simulink model "mdlref_basic"  (Simulink 7.8)
settings: Solver=FixedStepDiscrete  SolverMode=SingleTasking  StartTime=0.0  StopTime=10.0  FixedStep=0.1  RelTol=1e-3
settings Model: Creator=The MathWorks Inc.  LastModifiedBy=itoy  ExtModeAutoUpdateStatusClock=off
settings DataIOCC: SaveFormat=StructureWithTime  SignalLoggingName=logsOut
settings OptimizationCC: InlineParams=on  InlineInvariantSignals=on  InitFltsAndDblsToZero=on
settings DebuggingCC: SaveWithParameterizedLinksMsg=none  CheckExecutionContextPreStartOutputMsg=on  CheckExecutionContextRuntimeOutputMsg=on  SolverPrmCheckMsg=none  MultiTaskDSMMsg=warning  MultiTaskCondExecSysMsg=none  SigSpecEnsureSampleTimeMsg=none  FcnCallInpInsideContextMsg=Use local settings  StrictBusMsg=ErrorOnBusTreatedAsVector
settings HardwareCC: TargetHWDeviceType=32-bit Generic
settings ModelReferenceCC: UpdateModelReferenceTargets=IfOutOfDate  CheckModelReferenceTargetMessage=none
settings RTWCC: GenerateReport=on  ProcessScript=grt_make_rtw_hook  LaunchReport=on  IncludeERTFirstTime=on
settings CodeAppCC: MaxIdLength=100
settings GRTTargetCC: TargetFcnLib=ansi_tfl_tmw.mat

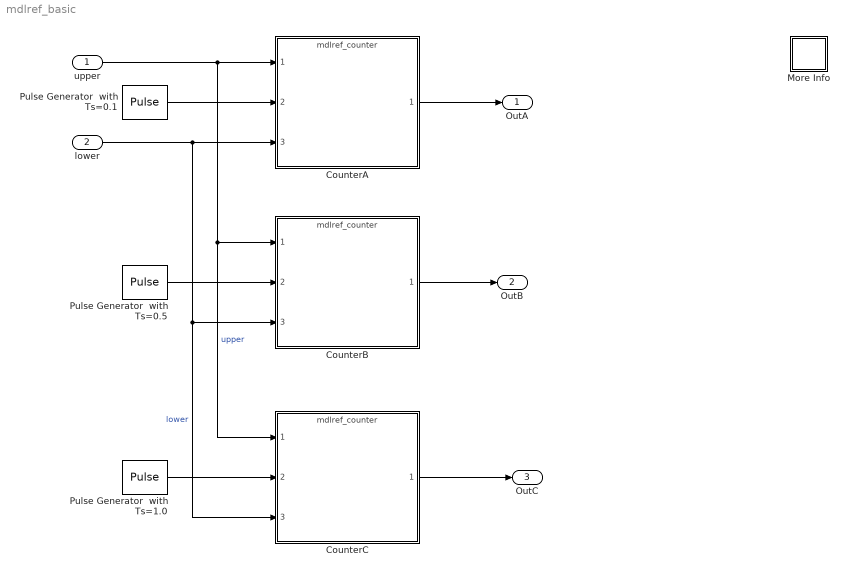
== system mdlref_basic ==
  upper : Inport
  lower : Inport  Port=2
  CounterA : ModelReference  ModelNameDialog=mdlref_counter  SimulationMode=Normal  ModelReferenceVersion=1.74  CopyOfModelName=mdlref_counter  DefaultDataLogging=off
  CounterB : ModelReference  ModelNameDialog=mdlref_counter  SimulationMode=Normal  ModelReferenceVersion=1.74  CopyOfModelName=mdlref_counter  DefaultDataLogging=off
  CounterC : ModelReference  ModelNameDialog=mdlref_counter  SimulationMode=Accelerator  ModelReferenceVersion=1.74  CopyOfModelName=mdlref_counter  DefaultDataLogging=off
  More Info : Subsystem
      settings: OpenFcn=showdemo(bdroot(gcb))
      mask Display: disp('?')
  Pulse Generator  with Ts=0.1 : DiscretePulseGenerator  SampleTime=0.1  VectorParams1D=off
  Pulse Generator  with Ts=0.5 : DiscretePulseGenerator  SampleTime=0.5
  Pulse Generator  with Ts=1.0 : DiscretePulseGenerator  SampleTime=1.0
  OutA : Outport
  OutB : Outport  Port=2
  OutC : Outport  Port=3
  wires:
  Pulse Generator  with Ts=0.1/1 -> CounterA/2
  Pulse Generator  with Ts=0.5/1 -> CounterB/2
  Pulse Generator  with Ts=1.0/1 -> CounterC/2
  upper/1 -> CounterA/1, CounterC/1, CounterB/1  "upper"
  lower/1 -> CounterA/3, CounterC/3, CounterB/3  "lower"
  CounterA/1 -> OutA/1
  CounterB/1 -> OutB/1
  CounterC/1 -> OutC/1

== system mdlref_basic/More Info ==
  note: Bus Block Demonstration
  note: This demonstration shows how signals may be grouped and ungrouped while
      | retaining their names.  In this demonstration, 5 signals are created and labelled
      | appropriately.  These signals are then mux'd together to create a bus of signals.
      | This bus of signals is then fed into the Bus Selector block.  Inside of the Bus
      | Selector block, the Pulse and Chirp signals are chosen to be output from the
      | original signal bus.
      |
      | It is possible to place a nest signal buses and then still retrieve the original signal
      | with its label.
